simulink model "Turbojet_thermodynamic_model"  (R2022b)
settings: Solver=VariableStepAuto  StartTime=0.0  StopTime=10.0  RelTol=1e-3
settings Model: Creator=carloshermoso  LastModifiedBy=carloshermoso

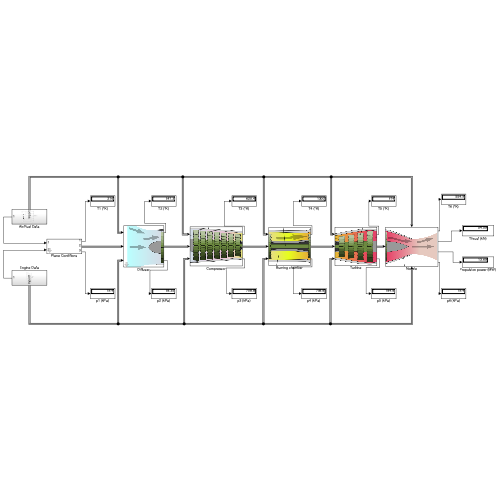
[thumbnail: Simulink's stored preview of the top-level diagram]
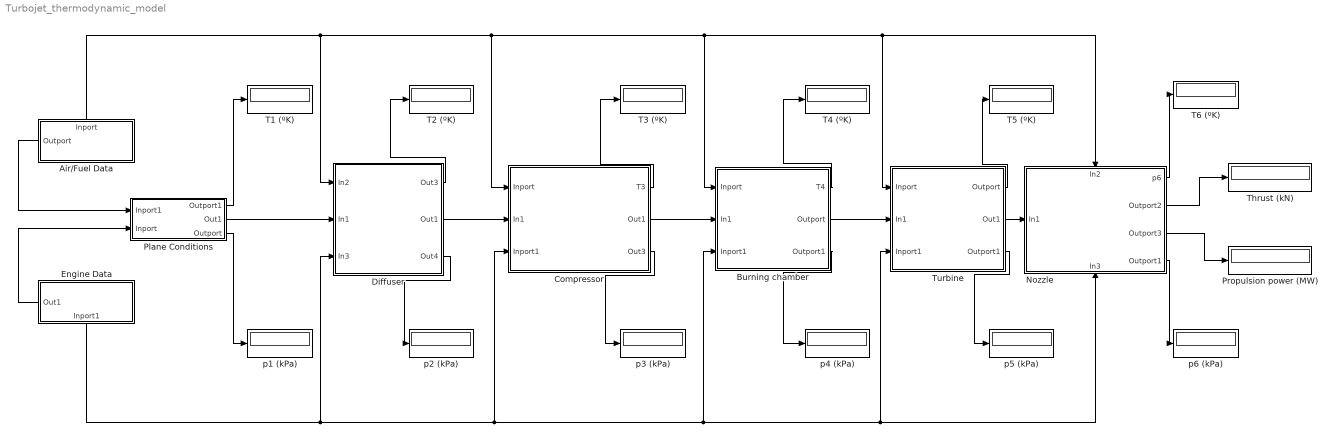
== system Turbojet_thermodynamic_model ==
  Air/Fuel Data : Subsystem
      settings: PortSchema="{\"entries\":[{\"content\":{\"sides\":[{\"content\":{\"connectorIds\":[]},\"type\":\"ConnectorPlacement.EquallySpacedRectSide\",\"uuid\":\"d6e062bf-ada7-4a1e-b6df-c6426bc39b21\"},{\"content\":{\"connectorIds\":[\"Out1\"],\"side\":\"RIGHT\"},\"type\":\"ConnectorPlacement.EquallySpacedRectSide\",\"uuid\":\"acf764d4-a69e-4191-a3e1-7fe9d6109cf5\"},{\"content\":{\"connectorIds\":[],\"side\":\"TOP\"},\"type\":\"ConnectorPlacement.EquallySpacedRectSide\",\"uuid\":\"bec8ee57-a4b3-43db-a6b3-4cc15b4852a0\"},{\"content\":{\"connectorIds\":[\"Out2\"],\"side\":\"BOTTOM\"},\"type\":\"ConnectorPlacement.EquallySpacedRectSide\",\"uuid\":\"7f13e328-219e-4693-98cf-3b1cd0a8a5be\"}]},\"type\":\"ConnectorPlacement.EquallySpacedConnector\",\"uuid\":\"57014837-09b0-4ebb-b744-19144ecb5663\"}],\"packageUris\":[\"http://schema.mathworks.com/mf0/Connector/R2020b\"],\"version\":\"1.0\"}"
  Burning chamber : Subsystem
      mask Display: image('/Users/carloshermoso/Carlos/Proyectos/Turbojet_Thermodynamic_Model/Images/combustion_chamber.svg.png'); % Use "Edit Image" on toolstrip to change.
  Compressor : Subsystem
      mask Display: image('/Users/carloshermoso/Carlos/Proyectos/Turbojet_Thermodynamic_Model/Images/compressor.png'); % Use "Edit Image" on toolstrip to change.
  Diffuser : Subsystem
      mask Display: image('/Users/carloshermoso/Carlos/Proyectos/Turbojet_Thermodynamic_Model/Images/Difusser.svg.png'); % Use "Edit Image" on toolstrip to change.
  Engine Data : Subsystem
      settings: PortSchema="{\"entries\":[{\"content\":{\"sides\":[{\"content\":{\"connectorIds\":[]},\"type\":\"ConnectorPlacement.EquallySpacedRectSide\",\"uuid\":\"73173a2b-a636-42b1-860e-34fdcb1be5d0\"},{\"content\":{\"connectorIds\":[\"Out1\"],\"side\":\"RIGHT\"},\"type\":\"ConnectorPlacement.EquallySpacedRectSide\",\"uuid\":\"63326185-9d6c-4a43-9cad-d00ff34d77a2\"},{\"content\":{\"connectorIds\":[\"Out2\"],\"side\":\"TOP\"},\"type\":\"ConnectorPlacement.EquallySpacedRectSide\",\"uuid\":\"3a1a641b-d100-428c-9669-633926674e4a\"},{\"content\":{\"connectorIds\":[],\"side\":\"BOTTOM\"},\"type\":\"ConnectorPlacement.EquallySpacedRectSide\",\"uuid\":\"9635eeb1-f07d-4fa9-a095-7355892f6a33\"}]},\"type\":\"ConnectorPlacement.EquallySpacedConnector\",\"uuid\":\"9cb7da85-f24a-463c-a355-af6d4b90e908\"}],\"packageUris\":[\"http://schema.mathworks.com/mf0/Connector/R2020b\"],\"version\":\"1.0\"}"
  Nozzle : Subsystem
      settings: PortSchema="{\"entries\":[{\"content\":{\"sides\":[{\"content\":{\"connectorIds\":[\"In1\"]},\"type\":\"ConnectorPlacement.EquallySpacedRectSide\",\"uuid\":\"23bdf9a9-d8c1-42a2-850a-9127a8d46717\"},{\"content\":{\"connectorIds\":[\"Out1\",\"Out2\",\"Out3\",\"Out4\"],\"side\":\"RIGHT\"},\"type\":\"ConnectorPlacement.EquallySpacedRectSide\",\"uuid\":\"6422cf2b-77d0-4167-ba79-4514bee64525\"},{\"content\":{\"connectorIds\":[\"In2\"],\"side\":\"TOP\"},\"type\":\"ConnectorPlacement.EquallySpacedRectSide\",\"uuid\":\"266aed2e-df5a-410c-8143-c8f252d426a4\"},{\"content\":{\"connectorIds\":[\"In3\"],\"side\":\"BOTTOM\"},\"type\":\"ConnectorPlacement.EquallySpacedRectSide\",\"uuid\":\"2513d2b4-1828-4861-ba40-ccbe0aed67c0\"}]},\"type\":\"ConnectorPlacement.EquallySpacedConnector\",\"uuid\":\"8007c893-1c38-411e-adb3-5360d1ea0823\"}],\"packageUris\":[\"http://schema.mathworks.com/mf0/Connector/R2020b\"],\"version\":\"1.0\"}"
      mask Display: image('/Users/carloshermoso/Carlos/Proyectos/Turbojet_Thermodynamic_Model/Images/nozzle.png'); % Use "Edit Image" on toolstrip to change.
  Plane Conditions : Subsystem  mask{w1=264.0, nozzle_style=Convergent-Divergent}
      mask prompts: w1 "Plane Speed (m/s)"; nozzle_style "Nozzle Style"
      mask TypeOptions nozzle_style: Convergent | Convergent-Divergent
  Propulsion power (MW) : Display
  T1 (ºK) : Display
  T2 (ºK) : Display
  T3 (ºK) : Display
  T4 (ºK) : Display
  T5 (ºK) : Display
  T6 (ºK) : Display
  Thrust (kN) : Display
  Turbine : Subsystem
      mask Display: image('/Users/carloshermoso/Carlos/Proyectos/Turbojet_Thermodynamic_Model/Images/Turbine.png'); % Use "Edit Image" on toolstrip to change.
  p1 (kPa) : Display
  p2 (kPa) : Display
  p3 (kPa) : Display
  p4 (kPa) : Display
  p5 (kPa) : Display
  p6 (kPa) : Display
  wires:
  Plane Conditions/2(Out1) -> Diffuser/2(In1)
  Engine Data/1(Out1) -> Plane Conditions/2(Inport)
  Air/Fuel Data/2(Inport) -> Diffuser/1(In2), Nozzle/2(In2), Turbine/1(Inport), Burning chamber/1(Inport), Compressor/1(Inport)
  Engine Data/2(Inport1) -> Diffuser/3(In3), Nozzle/3(In3), Turbine/3(Inport1), Burning chamber/3(Inport1), Compressor/3(Inport1)
  Diffuser/2(Out1) -> Compressor/2(In1)
  Air/Fuel Data/1(Outport) -> Plane Conditions/1(Inport1)
  Plane Conditions/1(Outport1) -> T1 (ºK)/1
  Plane Conditions/3(Outport) -> p1 (kPa)/1
  Diffuser/3(Out4) -> p2 (kPa)/1
  Diffuser/1(Out3) -> T2 (ºK)/1
  Compressor/3(Out3) -> p3 (kPa)/1
  Compressor/1(T3) -> T3 (ºK)/1
  Compressor/2(Out1) -> Burning chamber/2(In1)
  Burning chamber/1(T4) -> T4 (ºK)/1
  Burning chamber/3(Outport1) -> p4 (kPa)/1
  Burning chamber/2(Outport) -> Turbine/2(In1)
  Turbine/1(Outport) -> T5 (ºK)/1
  Turbine/2(Out1) -> Nozzle/1(In1)
  Turbine/3(Outport1) -> p5 (kPa)/1
  Nozzle/4(Outport1) -> p6 (kPa)/1
  Nozzle/1(p6) -> T6 (ºK)/1
  Nozzle/2(Outport2) -> Thrust (kN)/1
  Nozzle/3(Outport3) -> Propulsion power (MW)/1

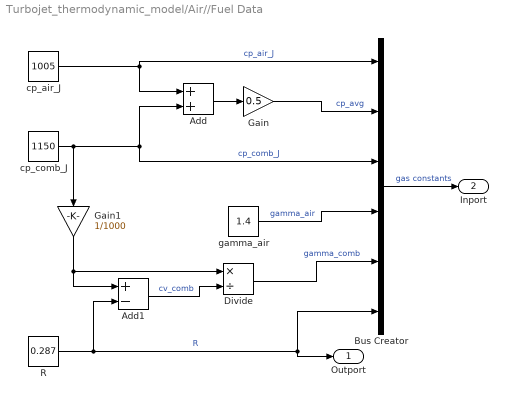
== system Turbojet_thermodynamic_model/Air//Fuel Data ==
  Add : Sum
  Add1 : Sum  Inputs=+-
  Bus Creator : BusCreator  Inputs=6
  Divide : Product  Inputs=*/
  Gain : Gain  Gain=0.5
  Gain1 : Gain  Gain=1/1000
  R : Constant  Value=0.287
  cp_air_J : Constant  Value=1005
  cp_comb_J : Constant  Value=1150
  gamma_air : Constant  Value=1.4
  Outport : Outport
  Inport : Outport  Port=2
  wires:
  gamma_air/1 -> Bus Creator/4  "gamma_air"
  R/1 -> Add1/2, Outport/1, Bus Creator/6  "R"
  cp_comb_J/1 -> Add/2, Bus Creator/3, Gain1/1  "cp_comb_J"
  Bus Creator/1 -> Inport/1  "gas constants"
  cp_air_J/1 -> Add/1, Bus Creator/1  "cp_air_J"
  Add/1 -> Gain/1
  Gain/1 -> Bus Creator/2  "cp_avg"
  Add1/1 -> Divide/2  "cv_comb"
  Divide/1 -> Bus Creator/5  "gamma_comb"
  Gain1/1 -> Divide/1, Add1/1

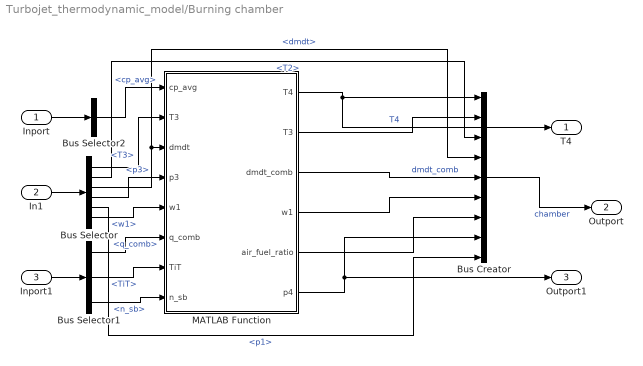
== system Turbojet_thermodynamic_model/Burning chamber ==
  Inport : Inport
  In1 : Inport  Port=2
  Inport1 : Inport  Port=3
  Bus Creator : BusCreator  Inputs=9
  Bus Selector : BusSelector  OutputSignals=T3,T2,dmdt,p3,p1,w1
  Bus Selector1 : BusSelector  OutputSignals=q_comb,TiT,n_sb
  Bus Selector2 : BusSelector  OutputSignals=cp_avg
  MATLAB Function : MATLAB Function  TreatAsAtomicUnit=on
  T4 : Outport
  Outport : Outport  Port=2
  Outport1 : Outport  Port=3
  wires:
  Bus Selector1/2 -> MATLAB Function/7(TiT)  "<TiT>"
  Bus Selector2/1 -> MATLAB Function/1(cp_avg)  "<cp_avg>"
  Bus Selector/1 -> MATLAB Function/2("T3 ")  "<T3>"
  In1/1 -> Bus Selector/1
  Inport1/1 -> Bus Selector1/1
  Bus Selector1/1 -> MATLAB Function/6(q_comb)  "<q_comb>"
  Bus Selector/3 -> MATLAB Function/3(dmdt), Bus Creator/4  "<dmdt>"
  Inport/1 -> Bus Selector2/1
  MATLAB Function/1(T4) -> T4/1, Bus Creator/1  "T4"
  MATLAB Function/3(dmdt_comb) -> Bus Creator/5  "dmdt_comb"
  Bus Selector/4 -> MATLAB Function/4(p3)  "<p3>"
  Bus Selector1/3 -> MATLAB Function/8(n_sb)  "<n_sb>"
  MATLAB Function/5(air_fuel_ratio) -> Bus Creator/7
  MATLAB Function/6(p4) -> Outport1/1, Bus Creator/8
  Bus Creator/1 -> Outport/1  "chamber"
  MATLAB Function/2(T3) -> Bus Creator/2
  Bus Selector/2 -> Bus Creator/3  "<T2>"
  Bus Selector/5 -> Bus Creator/9  "<p1>"
  Bus Selector/6 -> MATLAB Function/5("w1 ")  "<w1>"
  MATLAB Function/4(w1) -> Bus Creator/6

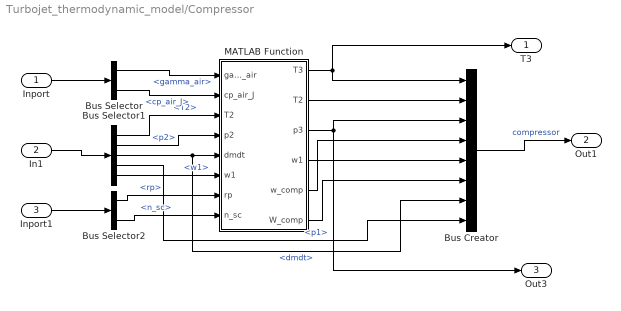
== system Turbojet_thermodynamic_model/Compressor ==
  Inport : Inport
  In1 : Inport  Port=2
  Inport1 : Inport  Port=3
  Bus Creator : BusCreator  Inputs=8
  Bus Selector : BusSelector  OutputSignals=gamma_air,cp_air_J
  Bus Selector1 : BusSelector  OutputSignals=T2,p2,dmdt,p1,w1
  Bus Selector2 : BusSelector  OutputSignals=rp,n_sc
  MATLAB Function : MATLAB Function  TreatAsAtomicUnit=on
  T3 : Outport
  Out1 : Outport  Port=2
  Out3 : Outport  Port=3
  wires:
  Inport1/1 -> Bus Selector2/1
  In1/1 -> Bus Selector1/1
  Inport/1 -> Bus Selector/1
  Bus Selector1/2 -> MATLAB Function/4(p2)  "<p2>"
  Bus Selector2/1 -> MATLAB Function/7(rp)  "<rp>"
  MATLAB Function/3(p3) -> Out3/1, Bus Creator/3
  Bus Selector/1 -> MATLAB Function/1(gamma_air)  "<gamma_air>"
  Bus Selector1/1 -> MATLAB Function/3("T2 ")  "<T2>"
  Bus Selector2/2 -> MATLAB Function/8(n_sc)  "<n_sc>"
  MATLAB Function/1(T3) -> Bus Creator/1, T3/1
  Bus Selector/2 -> MATLAB Function/2(cp_air_J)  "<cp_air_J>"
  Bus Selector1/3 -> Bus Creator/7, MATLAB Function/5(dmdt)  "<dmdt>"
  MATLAB Function/5(w_comp) -> Bus Creator/4
  MATLAB Function/6(W_comp) -> Bus Creator/6
  Bus Creator/1 -> Out1/1  "compressor"
  MATLAB Function/2(T2) -> Bus Creator/2
  Bus Selector1/4 -> Bus Creator/8  "<p1>"
  Bus Selector1/5 -> MATLAB Function/6("w1 ")  "<w1>"
  MATLAB Function/4(w1) -> Bus Creator/5

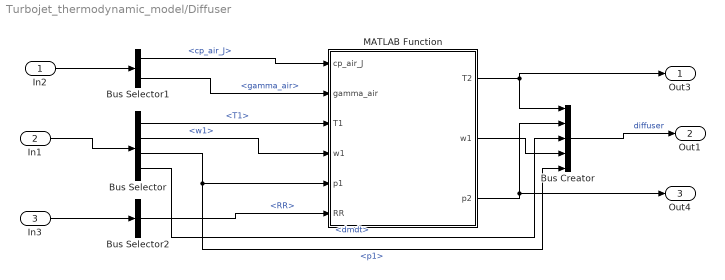
== system Turbojet_thermodynamic_model/Diffuser ==
  In2 : Inport
  In1 : Inport  Port=2
  In3 : Inport  Port=3
  Bus Creator : BusCreator  Inputs=5
  Bus Selector : BusSelector  OutputSignals=T1,w1,p1,dmdt
  Bus Selector1 : BusSelector  OutputSignals=cp_air_J,gamma_air
  Bus Selector2 : BusSelector  OutputSignals=RR
  MATLAB Function : MATLAB Function  TreatAsAtomicUnit=on
  Out3 : Outport
  Out1 : Outport  Port=2
  Out4 : Outport  Port=3
  wires:
  In1/1 -> Bus Selector/1
  Bus Selector/1 -> MATLAB Function/3(T1)  "<T1>"
  Bus Selector/2 -> MATLAB Function/4("w1 ")  "<w1>"
  In2/1 -> Bus Selector1/1
  Bus Selector1/1 -> MATLAB Function/1(cp_air_J)  "<cp_air_J>"
  In3/1 -> Bus Selector2/1
  Bus Selector1/2 -> MATLAB Function/2(gamma_air)  "<gamma_air>"
  Bus Selector2/1 -> MATLAB Function/6(RR)  "<RR>"
  Bus Selector/3 -> Bus Creator/5, MATLAB Function/5(p1)  "<p1>"
  MATLAB Function/3(p2) -> Bus Creator/2, Out4/1
  MATLAB Function/1(T2) -> Bus Creator/1, Out3/1
  Bus Creator/1 -> Out1/1  "diffuser"
  Bus Selector/4 -> Bus Creator/3  "<dmdt>"
  MATLAB Function/2(w1) -> Bus Creator/4

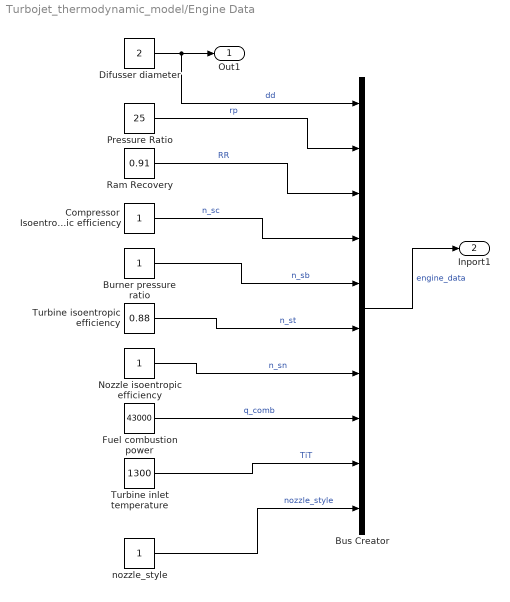
== system Turbojet_thermodynamic_model/Engine Data ==
  Burner pressure ratio : Constant
  Bus Creator : BusCreator  Inputs=10
  Compressor Isoentropic efficiency : Constant
  Difusser diameter : Constant  Value=2
  "Fuel combustion power " : Constant  Value=43000
  Nozzle isoentropic efficiency : Constant
  Pressure Ratio : Constant  Value=25
  Ram Recovery : Constant  Value=0.91
  Turbine inlet temperature : Constant  Value=1300
  Turbine isoentropic efficiency : Constant  Value=0.88
  nozzle_style : Constant
  Out1 : Outport
  Inport1 : Outport  Port=2
  wires:
  Pressure Ratio/1 -> Bus Creator/2  "rp"
  Ram Recovery/1 -> Bus Creator/3  "RR"
  Compressor Isoentropic efficiency/1 -> Bus Creator/4  "n_sc"
  Burner pressure ratio/1 -> Bus Creator/5  "n_sb"
  Turbine isoentropic efficiency/1 -> Bus Creator/6  "n_st"
  Nozzle isoentropic efficiency/1 -> Bus Creator/7  "n_sn"
  "Fuel combustion power "/1 -> Bus Creator/8  "q_comb"
  Difusser diameter/1 -> Bus Creator/1, Out1/1  "dd"
  Bus Creator/1 -> Inport1/1  "engine_data"
  Turbine inlet temperature/1 -> Bus Creator/9  "TiT"
  nozzle_style/1 -> Bus Creator/10  "nozzle_style"

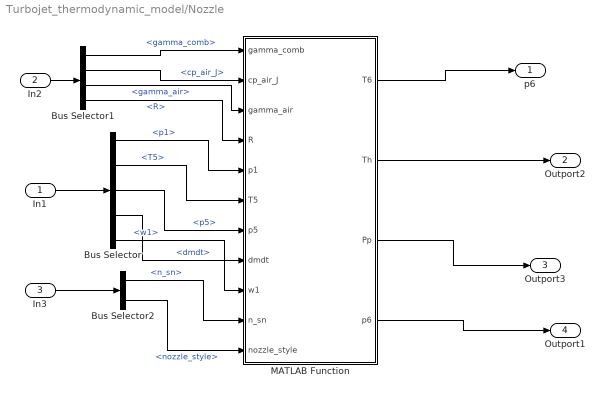
== system Turbojet_thermodynamic_model/Nozzle ==
  In1 : Inport
  In2 : Inport  Port=2
  In3 : Inport  Port=3
  Bus Selector : BusSelector  OutputSignals=p1,T5,p5,dmdt,w1
  Bus Selector1 : BusSelector  OutputSignals=gamma_comb,cp_air_J,gamma_air,R
  Bus Selector2 : BusSelector  OutputSignals=n_sn,nozzle_style
  MATLAB Function : MATLAB Function  TreatAsAtomicUnit=on
  p6 : Outport
  Outport2 : Outport  Port=2
  Outport3 : Outport  Port=3
  Outport1 : Outport  Port=4
  wires:
  In1/1 -> Bus Selector/1
  Bus Selector/1 -> MATLAB Function/5(p1)  "<p1>"
  MATLAB Function/4(p6) -> Outport1/1
  In2/1 -> Bus Selector1/1
  Bus Selector/2 -> MATLAB Function/6(T5)  "<T5>"
  Bus Selector/3 -> MATLAB Function/7(p5)  "<p5>"
  Bus Selector1/1 -> MATLAB Function/1(gamma_comb)  "<gamma_comb>"
  MATLAB Function/1(T6) -> p6/1
  Bus Selector1/2 -> MATLAB Function/2(cp_air_J)  "<cp_air_J>"
  In3/1 -> Bus Selector2/1
  Bus Selector2/1 -> MATLAB Function/10(n_sn)  "<n_sn>"
  Bus Selector1/3 -> MATLAB Function/3(gamma_air)  "<gamma_air>"
  Bus Selector1/4 -> MATLAB Function/4(R)  "<R>"
  Bus Selector2/2 -> MATLAB Function/11(nozzle_style)  "<nozzle_style>"
  Bus Selector/4 -> MATLAB Function/8(dmdt)  "<dmdt>"
  Bus Selector/5 -> MATLAB Function/9(w1)  "<w1>"
  MATLAB Function/2(Th) -> Outport2/1
  MATLAB Function/3(Pp) -> Outport3/1

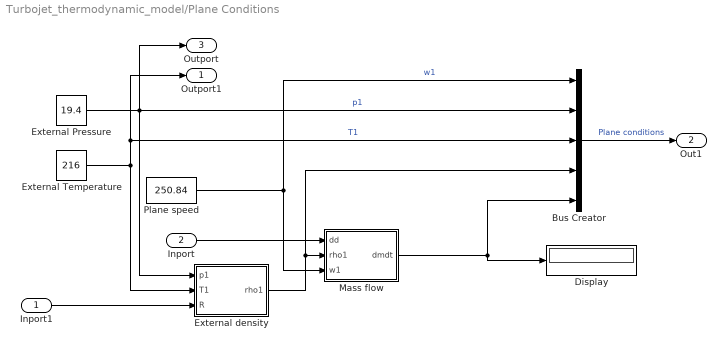
== system Turbojet_thermodynamic_model/Plane Conditions ==
  Inport1 : Inport
  Inport : Inport  Port=2
  Bus Creator : BusCreator  Inputs=5
  Display : Display
  External Pressure : Constant  Value=19.4
  External Temperature : Constant  Value=216
  External density : MATLAB Function  TreatAsAtomicUnit=on
  Mass flow : MATLAB Function  TreatAsAtomicUnit=on
  Plane speed : Constant  Value=250.84
  Outport1 : Outport
  Out1 : Outport  Port=2
  Outport : Outport  Port=3
  wires:
  External density/1(rho1) -> Mass flow/2(rho1), Bus Creator/4
  Inport/1 -> Mass flow/1(dd)
  Bus Creator/1 -> Out1/1  "Plane conditions"
  Plane speed/1 -> Mass flow/3(w1), Bus Creator/1  "w1"
  External Temperature/1 -> External density/2(T1), Outport1/1, Bus Creator/3  "T1"
  Inport1/1 -> External density/3(R)
  External Pressure/1 -> Outport/1, Bus Creator/2, External density/1(p1)  "p1"
  Mass flow/1(dmdt) -> Bus Creator/5, Display/1

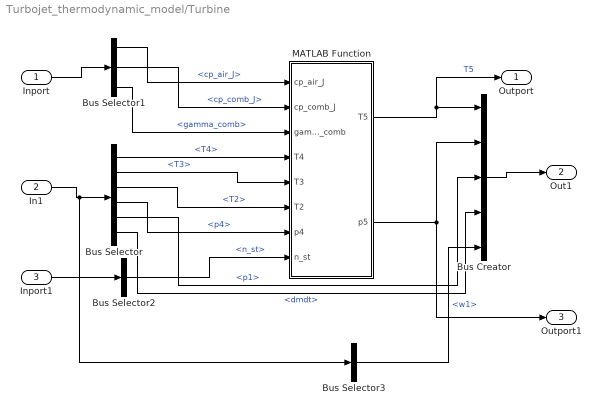
== system Turbojet_thermodynamic_model/Turbine ==
  Inport : Inport
  In1 : Inport  Port=2
  Inport1 : Inport  Port=3
  Bus Creator : BusCreator  Inputs=5
  Bus Selector : BusSelector  OutputSignals=T4,T3,T2,p4,p1,dmdt
  Bus Selector1 : BusSelector  OutputSignals=cp_air_J,cp_comb_J,gamma_comb
  Bus Selector2 : BusSelector  OutputSignals=n_st
  Bus Selector3 : BusSelector  OutputSignals=w1
  MATLAB Function : MATLAB Function  TreatAsAtomicUnit=on
  Outport : Outport
  Out1 : Outport  Port=2
  Outport1 : Outport  Port=3
  wires:
  In1/1 -> Bus Selector3/1, Bus Selector/1
  Bus Selector/1 -> MATLAB Function/4(T4)  "<T4>"
  Inport/1 -> Bus Selector1/1
  Bus Selector1/1 -> MATLAB Function/1(cp_air_J)  "<cp_air_J>"
  Bus Selector1/2 -> MATLAB Function/2(cp_comb_J)  "<cp_comb_J>"
  Bus Selector/2 -> MATLAB Function/5(T3)  "<T3>"
  Bus Selector/3 -> MATLAB Function/6(T2)  "<T2>"
  Inport1/1 -> Bus Selector2/1
  Bus Selector2/1 -> MATLAB Function/8(n_st)  "<n_st>"
  Bus Selector/4 -> MATLAB Function/7(p4)  "<p4>"
  Bus Selector1/3 -> MATLAB Function/3(gamma_comb)  "<gamma_comb>"
  MATLAB Function/2(p5) -> Outport1/1, Bus Creator/2
  MATLAB Function/1(T5) -> Bus Creator/1, Outport/1  "T5"
  Bus Creator/1 -> Out1/1
  Bus Selector/5 -> Bus Creator/3  "<p1>"
  Bus Selector/6 -> Bus Creator/4  "<dmdt>"
  Bus Selector3/1 -> Bus Creator/5  "<w1>"

== matlab function Turbojet_thermodynamic_model/Nozzle/MATLAB Function ==
  data: T6 output; Th output; Pp output; gamma_comb input; cp_air_J input; gamma_air input; R input; p1 input; p6 output; T5 input; p5 input; dmdt input; w1 input; n_sn input; nozzle_style input
function [T6,Th,Pp,p6]= fcn(gamma_comb,cp_air_J,gamma_air,R,p1,T5,p5,dmdt,w1,n_sn,nozzle_style)

p6 = p1;
T6s = T5*(p5/p6)^((1-gamma_comb)/gamma_comb);
w6s = (2*cp_air_J*(T5-T6s))^0.5;
w6 = n_sn^(0.5)*w6s;
T6 = T5-0.5*w6^2/cp_air_J;
c_T6 = (gamma_air*R*1000*T6)^(0.5);

Th = 0;
Pp = 0
if nozzle_style == 1
    w6 = c_T6;
    Th = dmdt*(w6-w1)/1000; %KN
    Pp = Th*w1/1000; %MW
end

== matlab function Turbojet_thermodynamic_model/Plane Conditions/Mass flow ==
  data: dd input; dmdt output; rho1 input; w1 input
function dmdt = fcn(dd,rho1,w1)

dmdt= (pi*(dd/2)^2)*rho1*w1;

== matlab function Turbojet_thermodynamic_model/Plane Conditions/External density ==
  data: p1 input; rho1 output; T1 input; R input
function rho1 = fcn(p1,T1,R)

rho1=p1/R/T1;

== matlab function Turbojet_thermodynamic_model/Diffuser/MATLAB Function ==
  data: cp_air_J input; gamma_air input; T1 input; T2 output; w1 output; w1 input; p2 output; p1 input; RR input
function [T2,w1,p2]= fcn(cp_air_J,gamma_air,T1,w1,p1,RR)

T2 = T1+0.5*w1^2/cp_air_J;
p2 = RR*p1*(T1/T2)^(gamma_air/(1-gamma_air));

== matlab function Turbojet_thermodynamic_model/Compressor/MATLAB Function ==
  data: T3 output; T2 output; gamma_air input; cp_air_J input; T2 input; p2 input; dmdt input; w1 input; p3 output; w1 output; rp input; n_sc input; w_comp output; W_comp output
function [T3, T2, p3,w1, w_comp, W_comp]= fcn(gamma_air, cp_air_J, T2, p2,dmdt,w1, rp, n_sc)

p3 = rp*p2;
T3s = T2*rp^((gamma_air-1)/gamma_air);
T3 = T2+(T3s-T2)/n_sc;
w_comp = (cp_air_J/1000)*(T2-T3); %kJ/kg
W_comp = (w_comp*dmdt)/1000; %MW

== matlab function Turbojet_thermodynamic_model/Burning chamber/MATLAB Function ==
  data: cp_avg input; T3 input; T4 output; T3 output; dmdt input; p3 input; w1 input; q_comb input; dmdt_comb output; w1 output; TiT input; n_sb input; air_fuel_ratio output; p4 output
function [T4,T3,dmdt_comb,w1,air_fuel_ratio, p4]= fcn(cp_avg,T3, dmdt,p3,w1,q_comb,TiT,n_sb)

T4 = TiT;
dmdt_comb = dmdt*(cp_avg/1000)*(T4-T3)/q_comb;
p4 = n_sb*p3;
air_fuel_ratio = dmdt/dmdt_comb;

== matlab function Turbojet_thermodynamic_model/Turbine/MATLAB Function ==
  data: cp_air_J input; cp_comb_J input; gamma_comb input; T4 input; T5 output; T3 input; T2 input; p4 input; n_st input; p5 output
function [T5,p5]= fcn(cp_air_J,cp_comb_J,gamma_comb,T4,T3,T2,p4,n_st)

T5 = T4-(cp_air_J/1000)/(cp_comb_J/1000)*(T3-T2);
T5s = T4-(T4-T5)/n_st;
p5 = p4*(T4/T5s)^(gamma_comb/(1-gamma_comb))
